simulink model "Nonlinear_Adaptive_controller"  (R2021a)
settings: Solver=VariableStepAuto  StartTime=0.0  StopTime=1000  RelTol=1e-3
libraries: simulink x2
settings Model: Creator=dell  LastModifiedBy=dell

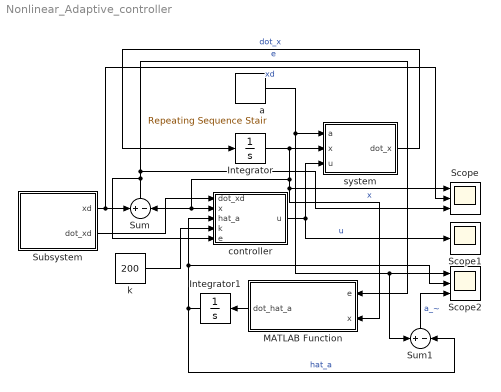
== system Nonlinear_Adaptive_controller ==
  Integrator : Integrator
  Integrator1 : Integrator
  MATLAB Function : MATLAB Function  TreatAsAtomicUnit=on
  Scope : Scope  NumInputPorts=3
  Scope1 : Scope
  Scope2 : Scope  NumInputPorts=3
  Subsystem : Subsystem
  Sum : Sum  Inputs=+-
  Sum1 : Sum  Inputs=+-
  a : simulink/Sources/Repeating Sequence Stair  OutValues=[3 1 4].'  tsamp=20  OutMin=[]  OutMax=[]  OutDataTypeStr=double  OutputDataTypeScalingMode=double  OutDataType=fixdt(0,8)  ConRadixGroup=Best Precision: Vector-wise  OutScaling=2^-12
  controller : MATLAB Function  TreatAsAtomicUnit=on
  k : Constant  Value=200
  system : MATLAB Function  TreatAsAtomicUnit=on
  wires:
  Integrator/1 -> Scope/1, MATLAB Function/2(x), Sum/2, controller/2(x), system/2(x)  "x"
  system/1(dot_x) -> Integrator/1  "dot_x"
  a/1 -> Sum1/1, Scope2/1, system/1(a)
  controller/1(u) -> Scope1/1, system/3(u)  "u"
  Subsystem/1(xd) -> Scope/2, Sum/1  "xd"
  Sum/1 -> Scope/3, MATLAB Function/1(e), controller/5(e)  "e"
  k/1 -> controller/4(k)
  Subsystem/2(dot_xd) -> controller/1(dot_xd)
  MATLAB Function/1(dot_hat_a) -> Integrator1/1
  Integrator1/1 -> Sum1/2, controller/3(hat_a), Scope2/2  "hat_a"
  Sum1/1 -> Scope2/3  "a_~"

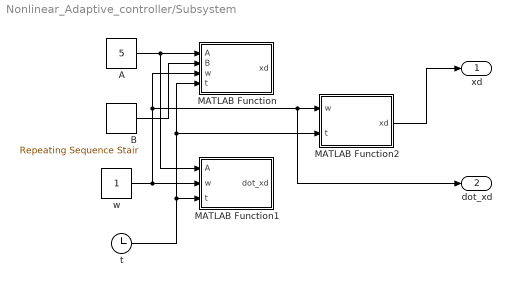
== system Nonlinear_Adaptive_controller/Subsystem ==
  A : Constant  Value=5
  B : simulink/Sources/Repeating Sequence Stair  OutValues=[5].'  tsamp=20  OutMin=[]  OutMax=[]  OutDataTypeStr=double  OutputDataTypeScalingMode=double  OutDataType=fixdt(0,8)  ConRadixGroup=Best Precision: Vector-wise  OutScaling=2^-12
  MATLAB Function : MATLAB Function  TreatAsAtomicUnit=on
  MATLAB Function1 : MATLAB Function  TreatAsAtomicUnit=on
  MATLAB Function2 : MATLAB Function  TreatAsAtomicUnit=on
  t : Clock
  w : Constant
  xd : Outport
  dot_xd : Outport  Port=2
  wires:
  A/1 -> MATLAB Function1/1(A), MATLAB Function/1(A)
  B/1 -> MATLAB Function/2(B)
  w/1 -> dot_xd/1, MATLAB Function2/1(w), MATLAB Function/3(w), MATLAB Function1/2(w)
  t/1 -> MATLAB Function2/2(t), MATLAB Function/4(t), MATLAB Function1/3(t)
  MATLAB Function2/1(xd) -> xd/1

== matlab function Nonlinear_Adaptive_controller/system ==
  data: a input; dot_x output; x input; u input
function dot_x = fcn(a,x,u)

dot_x = a*x^2+u;

== matlab function Nonlinear_Adaptive_controller/controller ==
  data: dot_xd input; u output; x input; hat_a input; k input; e input
function u = fcn(dot_xd,x,hat_a,k,e)

u = dot_xd-hat_a*x^2+k*e;

== matlab function Nonlinear_Adaptive_controller/MATLAB Function ==
  data: e input; dot_hat_a output; x input
function dot_hat_a = fcn(e,x)

dot_hat_a  = -e*x^2;

== matlab function Nonlinear_Adaptive_controller/Subsystem/MATLAB Function ==
  data: A input; xd output; B input; w input; t input
function xd = fcn(A,B,w,t)

xd = B+A*sin(w*t);

== matlab function Nonlinear_Adaptive_controller/Subsystem/MATLAB Function1 ==
  data: A input; dot_xd output; w input; t input
function dot_xd = fcn(A,w,t)

dot_xd = w*A*cos(w*t);

== matlab function Nonlinear_Adaptive_controller/Subsystem/MATLAB Function2 ==
  data: xd output; w input; t input
function xd = fcn(w,t)

xd = w*t;
